simulink model "verify_HeatExchanger_mdl"  (R2013b)
settings: Solver=ode45  StartTime=0.0  StopTime=3600  MaxStep=600  RelTol=1e-3
libraries: carnot x5
settings Model: Creator=drhf  LastModifiedBy=drhf
settings DataIOCC: SignalLoggingSaveFormat=ModelDataLogs  SignalLogging=off
settings OptimizationCC: ExpressionDepthLimit=2147483647
settings DebuggingCC: FcnCallInpInsideContextMsg=UseLocalSettings  StateNameClashWarn=warning
settings GRTTargetCC: CombineOutputUpdateFcns=off  GRTInterface=on

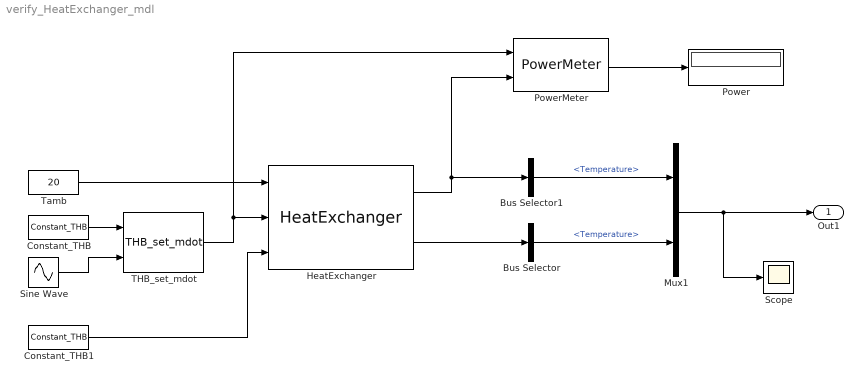
== system verify_HeatExchanger_mdl ==
  Bus Selector : BusSelector  OutputSignals=Temperature
  Bus Selector1 : BusSelector  OutputSignals=Temperature
  Constant_THB : carnot/Source/Simple/Constant_THB  t=40  mdot=50/3600  p=1e5  mID=No Pressure Drop  fluid=Water  mix=0  mix2=0  mix3=0  dia=0.02  hgt=0
  Constant_THB1 : carnot/Source/Simple/Constant_THB  t=10  mdot=500/3600  p=1e5  mID=No Pressure Drop  fluid=Water  mix=0  mix2=0  mix3=0  dia=0.02  hgt=0
  HeatExchanger : carnot/Source/Heat_Exchanger/HeatExchanger  flowtype=1  ua0=2000  uahot=[0.04 0]  uacold=[0.04 0]  ualoss=0  cap=10e3  linh=20  quah=10  linc=20  quac=10  t0=20
  Mux1 : Mux  Inputs=2
  Power : Display
  PowerMeter : carnot/Control/PowerMeter
  Scope : Scope
  Sine Wave : Sin  Amplitude=500/3600  Bias=400/3600  Frequency=2*pi/3600  SampleTime=0
  THB_set_mdot : carnot/Source/Simple/THB_set_mdot
  Tamb : Constant  Value=20
  Out1 : Outport  SampleTime=120
  wires:
  THB_set_mdot/1 -> PowerMeter/1, HeatExchanger/2
  PowerMeter/1 -> Power/1
  HeatExchanger/1 -> Bus Selector1/1, PowerMeter/2
  Constant_THB/1 -> THB_set_mdot/1
  Sine Wave/1 -> THB_set_mdot/2
  Constant_THB1/1 -> HeatExchanger/3
  Tamb/1 -> HeatExchanger/1
  HeatExchanger/2 -> Bus Selector/1
  Bus Selector/1 -> Mux1/2  "<Temperature>"
  Bus Selector1/1 -> Mux1/1  "<Temperature>"
  Mux1/1 -> Out1/1, Scope/1
